simulink model "My_Design"  (R2024b)
settings: Solver=ode23t  StartTime=0.0  StopTime=0.5  RelTol=1e-3
libraries: powerlib_extras x16, spsThreePhaseBreakerLib x7, spsSeriesRLCBranchLib x6, spsLinearTransformerLib x6, spsCurrentMeasurementLib x6, fuzblock x3, simulink_extras x3, spsThreePhaseFaultLib x3, spsThreePhasePISectionLineLib x2, spsThreePhaseSourceLib x1, spsThreePhaseSeriesRLCLoadLib x1, spsThreePhaseTransformerTwoWindingsLib x1
settings Model: PauseTimes=0.2999  Creator=Isaac  LastModifiedBy=oppon
settings SolverCC: AlgebraicLoopSolver=TrustRegion
settings DataIOCC: ReturnWorkspaceOutputs=off
settings DebuggingCC: UnconnectedInputMsg=warning  UnconnectedOutputMsg=warning  UnconnectedLineMsg=warning  ArithmeticOperatorsInVariantConditions=warning
settings ModelReferenceCC: EnableRefExpFcnMdlSchedulingChecks=on
settings SFSimCC: CustomCodeUndefinedFunction=UseInterfaceOnly
settings RTWCC: GPUComputeCapability=3.5

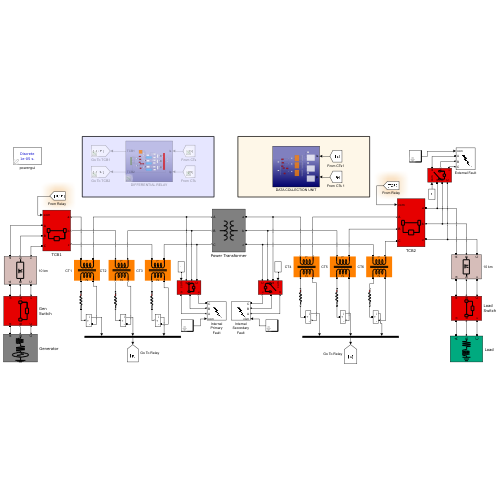
[thumbnail: Simulink's stored preview of the top-level diagram]
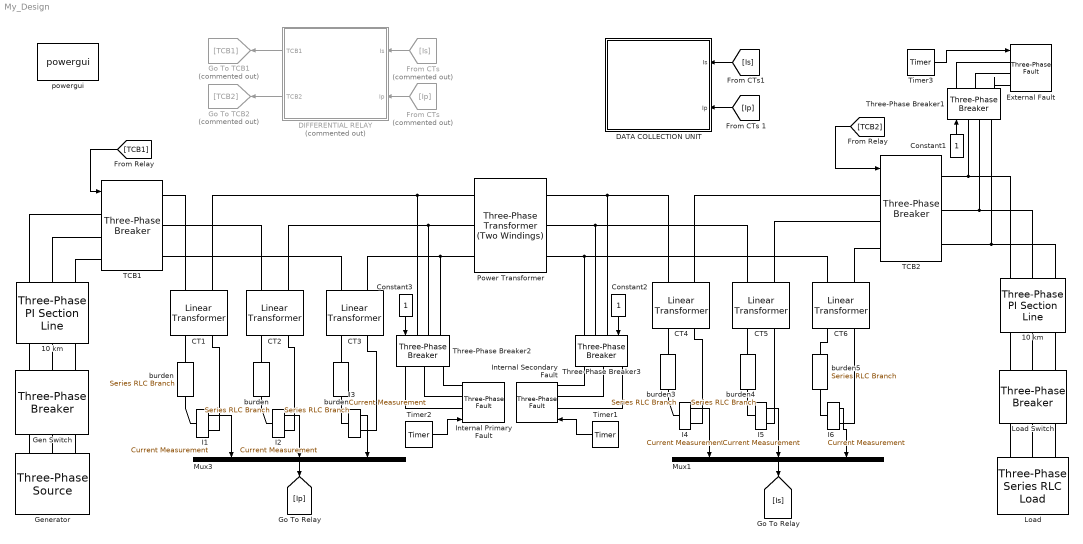
== system My_Design ==
  " burden " : spsSeriesRLCBranchLib/Series RLC Branch  LConnTagsString=__new0  RConnTagsString=__new0  BranchType=R  Resistance=1  Inductance=[]  SetiL0=off  InitialCurrent=0  Capacitance=[]  Setx0=off  InitialVoltage=0  Measurements=None
  10 km : spsThreePhasePISectionLineLib/Three-Phase PI Section Line  LConnTagsString=a|b|c  RConnTagsString=A|B|C  Length=10  Frequency=50  Resistances=[ 0.01273 0.3864]  Inductances="[ 0.9337e-3  4.1264e-3]"  Capacitances=[12.74e-9 7.751e-9]
  "10 km " : spsThreePhasePISectionLineLib/Three-Phase PI Section Line  LConnTagsString=a|b|c  RConnTagsString=A|B|C  Length=10  Frequency=50  Resistances=[ 0.01273 0.3864]  Inductances="[ 0.9337e-3  4.1264e-3]"  Capacitances=[12.74e-9 7.751e-9]
  CT1 : spsLinearTransformerLib/Linear Transformer  UNITS=pu  NominalPower=[ 25 50 ]  winding1=[12*(5/100) 0.001 0.04]  winding2=[5 0.001 0.04 ]  ThreeWindings=off  winding3=[ 315e3 0.002 0.08 ]  RmLm=[ 100 100 ]  Measurements=None  DataType=off
  CT2 : spsLinearTransformerLib/Linear Transformer  UNITS=pu  NominalPower=[ 25 50 ]  winding1=[12*(5/100) 0.001 0.04]  winding2=[5 0.001 0.04 ]  ThreeWindings=off  winding3=[ 315e3 0.002 0.08 ]  RmLm=[ 100 100 ]  Measurements=None  DataType=off
  CT3 : spsLinearTransformerLib/Linear Transformer  UNITS=pu  NominalPower=[ 25 50 ]  winding1=[12*(5/100) 0.001 0.04]  winding2=[5 0.001 0.04 ]  ThreeWindings=off  winding3=[ 315e3 0.002 0.08 ]  RmLm=[ 100 100 ]  Measurements=None  DataType=off
  CT4 : spsLinearTransformerLib/Linear Transformer  UNITS=pu  NominalPower=[ 25 50 ]  winding1=[14*(5/550) 0.001 0.04]  winding2=[5 0.001 0.04 ]  ThreeWindings=off  winding3=[ 315e3 0.002 0.08 ]  RmLm=[ 100 100 ]  Measurements=None  DataType=off
  CT5 : spsLinearTransformerLib/Linear Transformer  UNITS=pu  NominalPower=[ 25 50 ]  winding1=[14*(5/550) 0.001 0.04]  winding2=[5 0.001 0.04 ]  ThreeWindings=off  winding3=[ 315e3 0.002 0.08 ]  RmLm=[ 100 100 ]  Measurements=None  DataType=off
  CT6 : spsLinearTransformerLib/Linear Transformer  UNITS=pu  NominalPower=[ 25 50 ]  winding1=[14*(5/550) 0.001 0.04]  winding2=[5 0.001 0.04 ]  ThreeWindings=off  winding3=[ 315e3 0.002 0.08 ]  RmLm=[ 100 100 ]  Measurements=None  DataType=off
  Constant1 : Constant  OutDataTypeStr=boolean
  Constant2 : Constant  OutDataTypeStr=boolean
  Constant3 : Constant  OutDataTypeStr=boolean
  DATA COLLECTION UNIT : Subsystem
  DIFFERENTIAL RELAY : Subsystem  Commented=on
  External Fault : spsThreePhaseFaultLib/Three-Phase Fault  InitialStates=0  FaultA=on  FaultB=off  FaultC=off  GroundFault=on  SwitchTimes="[1/60  5/60]"  External=on  SwitchStatus=NaN  FaultResistance=0.001  GroundResistance=0.01  SnubberResistance=1e6  SnubberCapacitance=inf  Measurements=None
  From CTs : From  Commented=on  GotoTag=Is
  "From CTs " : From  Commented=on  GotoTag=Ip
  Gen Switch : spsThreePhaseBreakerLib/Three-Phase Breaker  InitialState=closed  SwitchA=off  SwitchB=off  SwitchC=off  SwitchTimes=[0.4/60 0.8/60 1/60 2.5/60]  External=off  BreakerResistance=0.001  SnubberResistance=1e6  SnubberCapacitance=inf  Measurements=None
  Generator : spsThreePhaseSourceLib/Three-Phase Source  InternalConnection=Yg  VoltagePhases=off  Voltage=161e3/sqrt(3)  PhaseAngle=0  Voltage_phases=[161e3 161e3 161e3]  PhaseAngles_phases=[0 -120 +120]  Frequency=50  NonIdealSource=on  SpecifyImpedance=on  Resistance=0.8929  Inductance=16.58e-3  ShortCircuitLevel=100e6  BaseVoltage=161e3/sqrt(3)  XRratio=2  BusType=swing  Pref=0  Qref=0  Prefabc=[10e3, 10e3, 10e3]  Qrefabc=[0, 0, 0]  Qmin=-inf  Qmax=inf
  Go To TCB1 : Goto  Commented=on  GotoTag=TCB1
  Go To TCB2 : Goto  Commented=on  GotoTag=TCB2
  I{1..6} (6 alike) : spsCurrentMeasurementLib/Current Measurement  Tag=PoWeRsYsTeMmEaSuReMeNt  PhasorSimulation=off  OutputType=Magnitude  PSBequivalent=0
      settings: AttributesFormatString=\n
  Internal Primary Fault : spsThreePhaseFaultLib/Three-Phase Fault  InitialStates=0  FaultA=on  FaultB=on  FaultC=on  GroundFault=off  SwitchTimes="[1/60  5/60]"  External=on  SwitchStatus=NaN  FaultResistance=0.001  GroundResistance=0.01  SnubberResistance=1e6  SnubberCapacitance=inf  Measurements=None
  Internal Secondary Fault : spsThreePhaseFaultLib/Three-Phase Fault  InitialStates=0  FaultA=on  FaultB=on  FaultC=on  GroundFault=on  SwitchTimes="[1/60  5/60]"  External=on  SwitchStatus=NaN  FaultResistance=0.001  GroundResistance=0.01  SnubberResistance=1e6  SnubberCapacitance=inf  Measurements=None
  Load : spsThreePhaseSeriesRLCLoadLib/Three-Phase Series RLC Load  LConnTagsString=A|B|C  Configuration=Y (grounded)  NominalVoltage=34.5e3  Vabc=[1e3 1e3 1e3]  Vabcp=[1e3 1e3 1e3]  NominalFrequency=50  UnbalancedPower=off  ActivePower=10e6  InductivePower=23e6  CapacitivePower=0  Pabc=[10e3 9e3 11e3]  QLabc=[100 90 110]  QCabc=[100 90 110]  Pabcp=[10e3 9e3 11e3]  QLabcp=[100 90 110]  QCabcp=[100 90 110]  Measurements=None  LoadType=constant Z
  Load Switch : spsThreePhaseBreakerLib/Three-Phase Breaker  InitialState=closed  SwitchA=off  SwitchB=off  SwitchC=off  SwitchTimes="[4/60  10/60]"  External=off  BreakerResistance=0.001  SnubberResistance=1e6  SnubberCapacitance=inf  Measurements=None
  Mux1 : Mux  Inputs=3
  Mux3 : Mux  Inputs=3
  Power Transformer : spsThreePhaseTransformerTwoWindingsLib/Three-Phase Transformer (Two Windings)  Winding1Connection=Yg  Winding2Connection=Yg  CoreType=Three-limb core (core-type)  SetSaturation=off  Hysteresis=off  DataFile='hysteresis'  SetInitialFlux=on  Measurements=All measurements (V I Fluxes)  UNITS=pu  NominalPower=[ 50e6 , 50 ]  Winding1=[1.61e+05 0.002 0.08]  Winding2=[34500 0.002 0.08]  Rm=500  Lm=1e6  L0=0.5  Saturation=[ 0,0 ; 0.015,1.2; 0.03,1.35; 0.06,1.5; 0.09,1.56; 0.12,1.572; 2.5e+12,1e+12]  InitialFluxes=[-0.291269118191543 0.0927265830204329 0.198559664112565]  BreakLoop=off  DiscreteSolver=Trapezoidal iterative  DataType=off  TransfoNumber=1
  TCB1 : spsThreePhaseBreakerLib/Three-Phase Breaker  InitialState=closed  SwitchA=off  SwitchB=off  SwitchC=off  SwitchTimes="[4/60  10/60]"  External=on  BreakerResistance=0.001  SnubberResistance=1e6  SnubberCapacitance=inf  Measurements=None
  TCB2 : spsThreePhaseBreakerLib/Three-Phase Breaker  InitialState=closed  SwitchA=off  SwitchB=off  SwitchC=off  SwitchTimes="[4/60  10/60]"  External=on  BreakerResistance=0.001  SnubberResistance=1e6  SnubberCapacitance=inf  Measurements=None
  Three-Phase Breaker1 : spsThreePhaseBreakerLib/Three-Phase Breaker  InitialState=open  SwitchA=on  SwitchB=on  SwitchC=on  SwitchTimes="[1/60  5/60]"  External=on  BreakerResistance=0.01  SnubberResistance=1e6  SnubberCapacitance=inf  Measurements=None
  Three-Phase Breaker2 : spsThreePhaseBreakerLib/Three-Phase Breaker  InitialState=closed  SwitchA=on  SwitchB=on  SwitchC=on  SwitchTimes="[1/60  5/60]"  External=on  BreakerResistance=0.01  SnubberResistance=1e6  SnubberCapacitance=inf  Measurements=None
  Three-Phase Breaker3 : spsThreePhaseBreakerLib/Three-Phase Breaker  InitialState=open  SwitchA=on  SwitchB=on  SwitchC=on  SwitchTimes="[1/60  5/60]"  External=on  BreakerResistance=0.01  SnubberResistance=1e6  SnubberCapacitance=inf  Measurements=None
  Timer1 : powerlib_extras/Control  Blocks/Timer  t=[0 0.3]  e=[0 1]
  Timer2 : powerlib_extras/Control  Blocks/Timer  t=[0 0.2]  e=[0 1]
  Timer3 : powerlib_extras/Control  Blocks/Timer  t=[0 0.4]  e=[0 1]
  burden{,3..5} (4 alike) : spsSeriesRLCBranchLib/Series RLC Branch  LConnTagsString=__new0  RConnTagsString=__new0  BranchType=R  Resistance=1  Inductance=[]  SetiL0=off  InitialCurrent=0  Capacitance=[]  Setx0=off  InitialVoltage=0  Measurements=None
  "burden " : spsSeriesRLCBranchLib/Series RLC Branch  LConnTagsString=__new0  RConnTagsString=__new0  BranchType=R  Resistance=1  Inductance=[]  SetiL0=off  InitialCurrent=0  Capacitance=[]  Setx0=off  InitialVoltage=0  Measurements=None
  powergui : sps_lib/powergui  Priority=1  SimulationMode=Discrete  SampleTime=1e-5  frequency=50  Iterations=50  frequencyindice=50  Pbase=100e6  ErrMax=1e-4  UnitsV=kV  UnitsW=MW  buscounter=0  FunctionMessages=off  echomessages=off  EnableUseOfTLC=off  CurrentSourceSwitches=off  DisableSnubberDevices=off  DisableRonSwitches=off  DisableVfSwitches=off  DisplayEquations=off  AutomaticDiscreteSolvers=off  SolverType=Tustin/Backward Euler (TBE)  Interpol=off  ExternalGateDelay=off  methode=off  Ts=100  x0status=blocks  SPID=off  SwTol=0  HookPort=off  NonlinearTolerance=1e-4  nMaxIteration=100  ContinueOnMaxIteration=off  RestoreLinks=warning  ResistiveCurrentMeasurement=off  Frange=[0:2:500]  Ylog=off  Xlog=on  ShowGrid=off  save=off  variable=ZData  structure=0  ZoomFFT=on  StartTime=0.0  cycles=1  DisplayStyle=1  fundamental=60  FreqAxis=off  MaxFrequency=1000  frequencyindicesteady=1  RmsSteady=1  display=off
  wires:
  Constant3/1 -> Three-Phase Breaker2/1
  Timer3/1 -> External Fault/1
  I4/1 -> Mux1/1
  Constant1/1 -> Three-Phase Breaker1/1
  I1/1 -> Mux3/1
  Mux1/1 -> [Is]
  [TCB1] -> TCB1/1
  Mux3/1 -> [Ip]
  I6/1 -> Mux1/3
  Timer1/1 -> Internal Secondary Fault/1
  [TCB2] -> TCB2/1
  I2/1 -> Mux3/2
  Timer2/1 -> Internal Primary Fault/1
  I5/1 -> Mux1/2
  Constant2/1 -> Three-Phase Breaker3/1
  DIFFERENTIAL RELAY/1(TCB1) -> Go To TCB1/1
  I3/1 -> Mux3/3
  "From CTs "/1 -> DIFFERENTIAL RELAY/2(Ip)
  From CTs/1 -> DIFFERENTIAL RELAY/1(Is)
  DIFFERENTIAL RELAY/2(TCB2) -> Go To TCB2/1
  [Is] -> DATA COLLECTION UNIT/1(Is)
  [Ip] -> DATA COLLECTION UNIT/2(Ip)
  connections:
  Three-Phase Breaker1/LConn1 -- TCB2/RConn1 -- "10 km "/LConn1
  Power Transformer/RConn1 -- CT4/LConn2 -- Three-Phase Breaker3/LConn1
  Three-Phase Breaker2/LConn1 -- CT1/LConn1 -- Power Transformer/LConn1
  Power Transformer/RConn3 -- CT6/LConn2 -- Three-Phase Breaker3/LConn3
  Three-Phase Breaker2/LConn2 -- CT2/LConn1 -- Power Transformer/LConn2
  "10 km "/LConn2 -- TCB2/RConn2 -- Three-Phase Breaker1/LConn2
  "10 km "/LConn3 -- TCB2/RConn3 -- Three-Phase Breaker1/LConn3
  Power Transformer/RConn2 -- CT5/LConn2 -- Three-Phase Breaker3/LConn2
  Three-Phase Breaker2/LConn3 -- CT3/LConn1 -- Power Transformer/LConn3
  10 km/RConn2 -- TCB1/LConn2
  Three-Phase Breaker1/RConn2 -- External Fault/LConn2
  10 km/RConn3 -- TCB1/LConn3
  burden/RConn1 -- I1/LConn1
  Three-Phase Breaker3/RConn3 -- Internal Secondary Fault/LConn3
  CT3/LConn2 -- TCB1/RConn3
  burden3/LConn1 -- CT4/RConn2
  Three-Phase Breaker1/RConn3 -- External Fault/LConn3
  CT4/LConn1 -- TCB2/LConn1
  I6/RConn1 -- CT6/RConn1
  burden4/LConn1 -- CT5/RConn2
  burden5/RConn1 -- I6/LConn1
  burden5/LConn1 -- CT6/RConn2
  CT6/LConn1 -- TCB2/LConn3
  CT2/LConn2 -- TCB1/RConn2
  "10 km "/RConn1 -- Load Switch/LConn1
  "burden "/LConn1 -- CT2/RConn2
  Gen Switch/LConn1 -- Generator/RConn1
  I1/RConn1 -- CT1/RConn1
  I3/RConn1 -- CT3/RConn1
  I4/RConn1 -- CT4/RConn1
  "10 km "/RConn2 -- Load Switch/LConn2
  "10 km "/RConn3 -- Load Switch/LConn3
  Three-Phase Breaker2/RConn3 -- Internal Primary Fault/LConn3
  " burden "/LConn1 -- CT3/RConn2
  Three-Phase Breaker2/RConn2 -- Internal Primary Fault/LConn2
  burden/LConn1 -- CT1/RConn2
  Load/LConn3 -- Load Switch/RConn3
  10 km/LConn3 -- Gen Switch/RConn3
  Gen Switch/LConn3 -- Generator/RConn3
  Gen Switch/LConn2 -- Generator/RConn2
  10 km/LConn1 -- Gen Switch/RConn1
  10 km/RConn1 -- TCB1/LConn1
  Load Switch/RConn1 -- Load/LConn1
  Three-Phase Breaker1/RConn1 -- External Fault/LConn1
  CT5/RConn1 -- I5/RConn1
  burden3/RConn1 -- I4/LConn1
  Three-Phase Breaker3/RConn1 -- Internal Secondary Fault/LConn1
  burden4/RConn1 -- I5/LConn1
  "burden "/RConn1 -- I2/LConn1
  Three-Phase Breaker3/RConn2 -- Internal Secondary Fault/LConn2
  CT5/LConn1 -- TCB2/LConn2
  Load/LConn2 -- Load Switch/RConn2
  Three-Phase Breaker2/RConn1 -- Internal Primary Fault/LConn1
  " burden "/RConn1 -- I3/LConn1
  10 km/LConn2 -- Gen Switch/RConn2
  CT2/RConn1 -- I2/RConn1
  CT1/LConn2 -- TCB1/RConn1

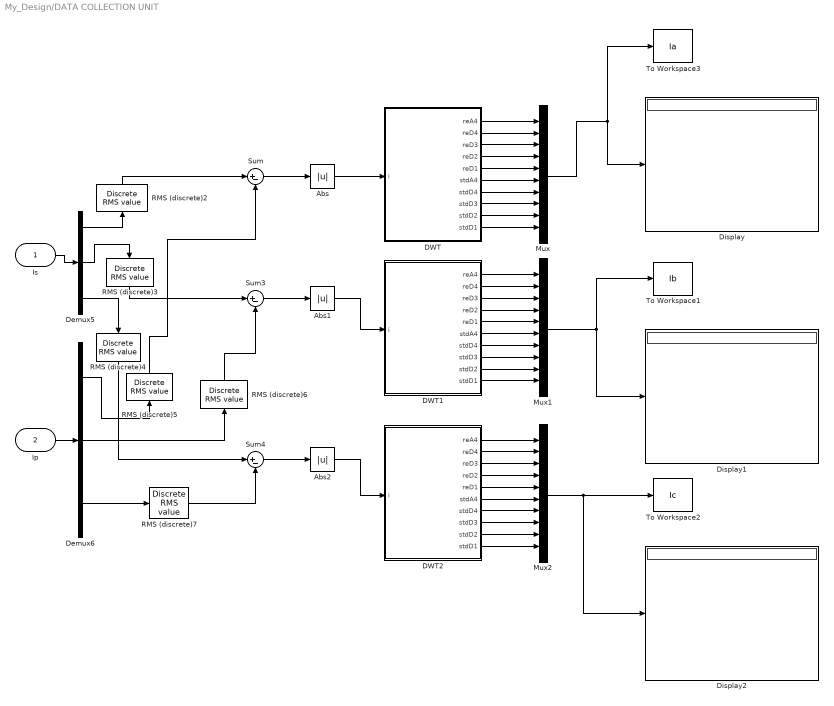
== system My_Design/DATA COLLECTION UNIT ==
  Is : Inport
  Ip : Inport  Port=2
  Abs : Abs  SaturateOnIntegerOverflow=off
  Abs1 : Abs  SaturateOnIntegerOverflow=off
  Abs2 : Abs  SaturateOnIntegerOverflow=off
  DWT : MATLAB Function  TreatAsAtomicUnit=on
  DWT1 : MATLAB Function  TreatAsAtomicUnit=on
  DWT2 : MATLAB Function  TreatAsAtomicUnit=on
  Demux5 : Demux  Outputs=3
  Demux6 : Demux  Outputs=3
  Display : Display
  Display1 : Display
  Display2 : Display
  Mux : Mux  Inputs=10
  Mux1 : Mux  Inputs=10
  Mux2 : Mux  Inputs=10
  RMS (discrete){2..7} (6 alike) : powerlib_extras/Discrete Measurements/Discrete  RMS value  Freq=50  Mag_Init=0  Ts=0.001
  Sum : Sum  Inputs=|+-
  Sum3 : Sum  Inputs=|+-
  Sum4 : Sum  Inputs=|+-
  To Workspace1 : ToWorkspace  VariableName=Ib  SampleTime=-1
      settings: Save2DSignal=2-D array (concatenate along first dimension)
  To Workspace2 : ToWorkspace  VariableName=Ic  SampleTime=-1
      settings: Save2DSignal=2-D array (concatenate along first dimension)
  To Workspace3 : ToWorkspace  VariableName=Ia  SampleTime=-1
      settings: Save2DSignal=2-D array (concatenate along first dimension)
  wires:
  Demux6/1 -> RMS (discrete)5/1
  Demux5/2 -> RMS (discrete)3/1
  Demux6/2 -> RMS (discrete)6/1
  Demux5/1 -> RMS (discrete)2/1
  Demux5/3 -> RMS (discrete)4/1
  Demux6/3 -> RMS (discrete)7/1
  Is/1 -> Demux5/1
  Ip/1 -> Demux6/1
  RMS (discrete)2/1 -> Sum/1
  RMS (discrete)5/1 -> Sum/2
  RMS (discrete)3/1 -> Sum3/1
  RMS (discrete)4/1 -> Sum4/1
  RMS (discrete)6/1 -> Sum3/2
  RMS (discrete)7/1 -> Sum4/2
  Sum/1 -> Abs/1
  Sum3/1 -> Abs1/1
  Sum4/1 -> Abs2/1
  Abs/1 -> DWT/1(i)
  DWT/1(reA4) -> Mux/1
  DWT/2(reD4) -> Mux/2
  DWT/3(reD3) -> Mux/3
  DWT/4(reD2) -> Mux/4
  DWT/5(reD1) -> Mux/5
  DWT/6(stdA4) -> Mux/6
  DWT/7(stdD4) -> Mux/7
  DWT/8(stdD3) -> Mux/8
  DWT/9(stdD2) -> Mux/9
  DWT/10(stdD1) -> Mux/10
  Mux/1 -> To Workspace3/1, Display/1
  DWT1/6(stdA4) -> Mux1/6
  DWT1/5(reD1) -> Mux1/5
  DWT1/2(reD4) -> Mux1/2
  DWT1/1(reA4) -> Mux1/1
  DWT1/4(reD2) -> Mux1/4
  DWT1/10(stdD1) -> Mux1/10
  DWT1/9(stdD2) -> Mux1/9
  DWT1/3(reD3) -> Mux1/3
  DWT1/8(stdD3) -> Mux1/8
  DWT1/7(stdD4) -> Mux1/7
  DWT2/6(stdA4) -> Mux2/6
  DWT2/5(reD1) -> Mux2/5
  DWT2/2(reD4) -> Mux2/2
  DWT2/1(reA4) -> Mux2/1
  DWT2/4(reD2) -> Mux2/4
  DWT2/10(stdD1) -> Mux2/10
  DWT2/9(stdD2) -> Mux2/9
  DWT2/3(reD3) -> Mux2/3
  DWT2/8(stdD3) -> Mux2/8
  DWT2/7(stdD4) -> Mux2/7
  Abs2/1 -> DWT2/1(i)
  Abs1/1 -> DWT1/1(i)
  Mux2/1 -> Display2/1, To Workspace2/1
  Mux1/1 -> Display1/1, To Workspace1/1

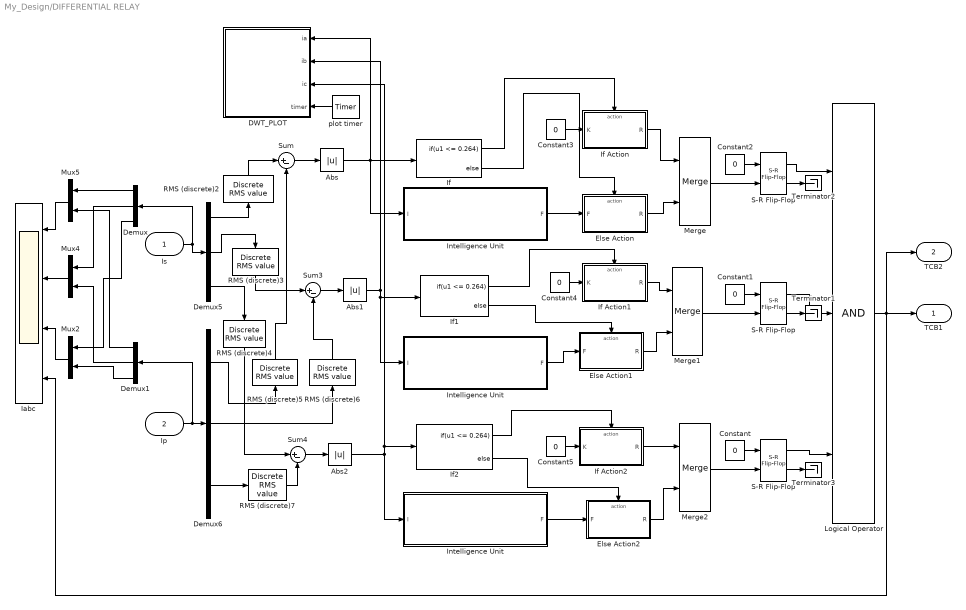
== system My_Design/DIFFERENTIAL RELAY ==
  Is : Inport
  Ip : Inport  Port=2
  " Logical Operator" : Logic  Inputs=3  AllPortsSameDT=off  OutDataTypeStr=boolean
  Abs : Abs  SaturateOnIntegerOverflow=off
  Abs1 : Abs  SaturateOnIntegerOverflow=off
  Abs2 : Abs  SaturateOnIntegerOverflow=off
  Constant{,1..5} (6 alike) : Constant  Value=0  OutDataTypeStr=boolean
  DWT_PLOT : MATLAB Function  TreatAsAtomicUnit=on
  Demux{,1,5..6} (4 alike) : Demux  Outputs=3
  Else Action : Subsystem  TreatAsAtomicUnit=on
  Else Action1 : Subsystem  TreatAsAtomicUnit=on
  Else Action2 : Subsystem  TreatAsAtomicUnit=on
  Iabc : Scope  NumInputPorts=4
  If : If  IfExpression=u1 <= 0.264
  If Action : Subsystem  TreatAsAtomicUnit=on
  If Action1 : Subsystem  TreatAsAtomicUnit=on
  If Action2 : Subsystem  TreatAsAtomicUnit=on
  If1 : If  IfExpression=u1 <= 0.264
  If2 : If  IfExpression=u1 <= 0.264
  Intelligence Unit : Subsystem
  "Intelligence Unit " : Subsystem
  "Intelligence Unit  " : Subsystem
  Merge : Merge
  Merge1 : Merge
  Merge2 : Merge
  Mux2 : Mux  Inputs=2
  Mux4 : Mux  Inputs=2
  Mux5 : Mux  Inputs=2
  RMS (discrete){2..7} (6 alike) : powerlib_extras/Discrete Measurements/Discrete  RMS value  Freq=50  Mag_Init=0  Ts=0.001
  "S-R Flip-Flop " : simulink_extras/Flip Flops/S-R Flip-Flop  initial_condition=1
  "S-R Flip-Flop  " : simulink_extras/Flip Flops/S-R Flip-Flop  initial_condition=1
  S-R Flip-Flop : simulink_extras/Flip Flops/S-R Flip-Flop  initial_condition=1
  Sum : Sum  Inputs=|+-
  Sum3 : Sum  Inputs=|+-
  Sum4 : Sum  Inputs=|+-
  Terminator1 : Terminator
  Terminator2 : Terminator
  Terminator3 : Terminator
  plot timer : powerlib_extras/Control  Blocks/Timer  t=[0 0.299999999999]  e=[0 1]
  TCB1 : Outport  VectorParamsAs1DForOutWhenUnconnected=off
  TCB2 : Outport  Port=2  VectorParamsAs1DForOutWhenUnconnected=off
  wires:
  "S-R Flip-Flop  "/1 -> " Logical Operator"/3
  Constant/1 -> "S-R Flip-Flop  "/1
  "S-R Flip-Flop  "/2 -> Terminator3/1
  "S-R Flip-Flop "/2 -> Terminator1/1
  Constant1/1 -> "S-R Flip-Flop "/1
  Constant2/1 -> S-R Flip-Flop/1
  S-R Flip-Flop/2 -> Terminator2/1
  S-R Flip-Flop/1 -> " Logical Operator"/1
  "S-R Flip-Flop "/1 -> " Logical Operator"/2
  Demux6/1 -> RMS (discrete)5/1
  Demux5/2 -> RMS (discrete)3/1
  Demux6/2 -> RMS (discrete)6/1
  Demux5/1 -> RMS (discrete)2/1
  Demux5/3 -> RMS (discrete)4/1
  Demux6/3 -> RMS (discrete)7/1
  If1/1 -> If Action1/Action
  If/2 -> Else Action/Action
  If1/2 -> Else Action1/Action
  Intelligence Unit/1(F) -> Else Action/1(F)
  Else Action/1(R) -> Merge/2
  If Action/1(R) -> Merge/1
  Merge/1 -> S-R Flip-Flop/2
  Merge1/1 -> "S-R Flip-Flop "/2
  Merge2/1 -> "S-R Flip-Flop  "/2
  Constant3/1 -> If Action/1(K)
  Constant4/1 -> If Action1/1(K)
  Demux1/2 -> Mux4/2
  Demux1/3 -> Mux2/2
  Mux5/1 -> Iabc/1
  Demux1/1 -> Mux5/2
  Demux/1 -> Mux5/1
  Mux2/1 -> Iabc/3
  Demux/2 -> Mux4/1
  Mux4/1 -> Iabc/2
  Demux/3 -> Mux2/1
  Is/1 -> Demux/1, Demux5/1
  " Logical Operator"/1 -> Iabc/4, TCB2/1, TCB1/1
  Ip/1 -> Demux1/1, Demux6/1
  RMS (discrete)2/1 -> Sum/1
  RMS (discrete)5/1 -> Sum/2
  RMS (discrete)3/1 -> Sum3/1
  RMS (discrete)4/1 -> Sum4/1
  RMS (discrete)6/1 -> Sum3/2
  RMS (discrete)7/1 -> Sum4/2
  Sum/1 -> Abs/1
  Abs/1 -> DWT_PLOT/1(ia), Intelligence Unit/1(I), If/1
  Sum3/1 -> Abs1/1
  Abs1/1 -> "Intelligence Unit "/1(I), If1/1, DWT_PLOT/2(ib)
  Sum4/1 -> Abs2/1
  Abs2/1 -> DWT_PLOT/3(ic), If2/1, "Intelligence Unit  "/1(I)
  If/1 -> If Action/Action
  "Intelligence Unit  "/1(F) -> Else Action2/1(F)
  If Action1/1(R) -> Merge1/1
  "Intelligence Unit "/1(F) -> Else Action1/1(F)
  Else Action1/1(R) -> Merge1/2
  Constant5/1 -> If Action2/1(K)
  If Action2/1(R) -> Merge2/1
  If2/1 -> If Action2/Action
  If2/2 -> Else Action2/Action
  Else Action2/1(R) -> Merge2/2
  plot timer/1 -> DWT_PLOT/4(timer)

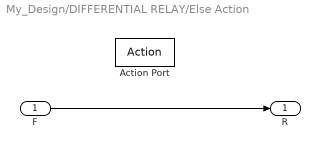
== system My_Design/DIFFERENTIAL RELAY/Else Action ==
  F : Inport
  Action Port : ActionPort  ActionPortLabel=else
  R : Outport  VectorParamsAs1DForOutWhenUnconnected=off
  wires:
  F/1 -> R/1

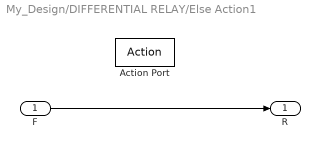
== system My_Design/DIFFERENTIAL RELAY/Else Action1 ==
  F : Inport
  Action Port : ActionPort  ActionPortLabel=else
  R : Outport  VectorParamsAs1DForOutWhenUnconnected=off
  wires:
  F/1 -> R/1

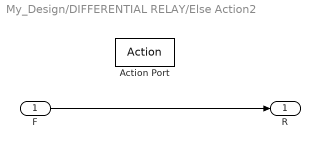
== system My_Design/DIFFERENTIAL RELAY/Else Action2 ==
  F : Inport
  Action Port : ActionPort  ActionPortLabel=else
  R : Outport  VectorParamsAs1DForOutWhenUnconnected=off
  wires:
  F/1 -> R/1

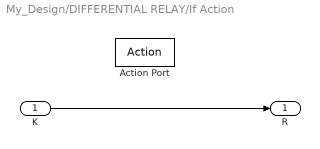
== system My_Design/DIFFERENTIAL RELAY/If Action ==
  K : Inport
  Action Port : ActionPort  ActionPortLabel=if(u1 <= 0.264)
  R : Outport
  wires:
  K/1 -> R/1

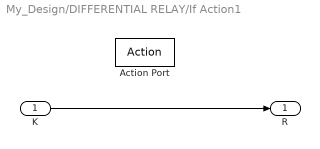
== system My_Design/DIFFERENTIAL RELAY/If Action1 ==
  K : Inport
  Action Port : ActionPort  ActionPortLabel=if(u1 <= 0.264)
  R : Outport
  wires:
  K/1 -> R/1

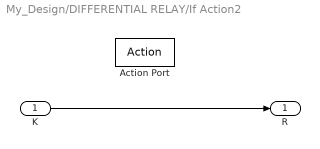
== system My_Design/DIFFERENTIAL RELAY/If Action2 ==
  K : Inport
  Action Port : ActionPort  ActionPortLabel=if(u1 <= 0.264)
  R : Outport
  wires:
  K/1 -> R/1

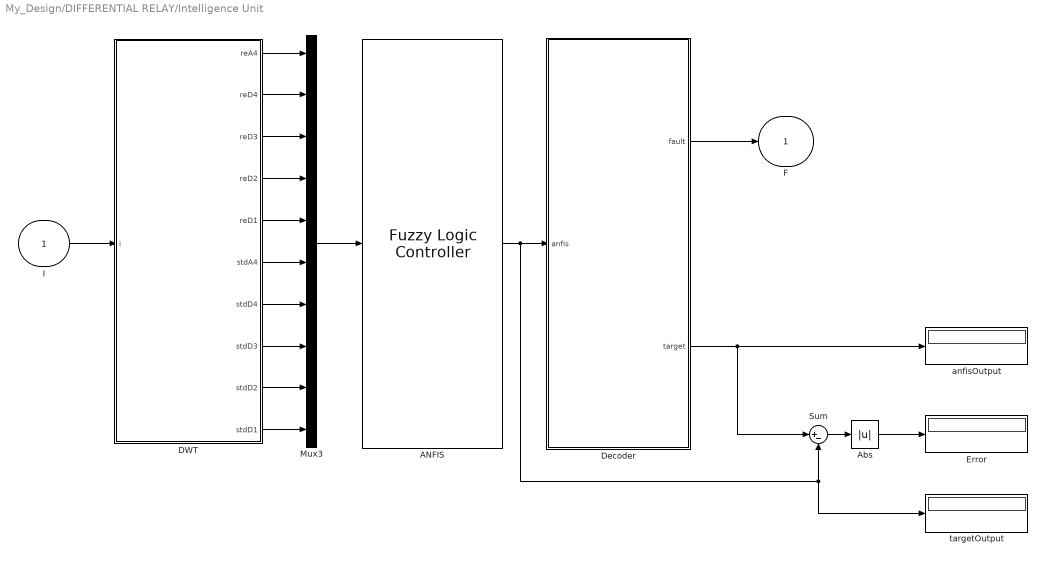
== system My_Design/DIFFERENTIAL RELAY/Intelligence Unit ==
  I : Inport
  ANFIS : fuzblock/Fuzzy Logic  Controller  FIS='classifier.fis'  OutputSampleNumber=101  DataType=double  FuzzifiedInputs=off  RuleFiringStrengths=off  RuleOutputs=off  AggregatedOutputs=off  SimulateUsing=Interpreted execution  OutOfRangeInputValueMessage=warning  NoRuleFiredMessage=warning  EmptyOutputFuzzySetMessage=warning
  Abs : Abs  SaturateOnIntegerOverflow=off
  DWT : MATLAB Function  TreatAsAtomicUnit=on
  Decoder : MATLAB Function  TreatAsAtomicUnit=on
  Error : Display
  Mux3 : Mux  Inputs=10
  Sum : Sum  Inputs=|+-
  anfisOutput : Display
  targetOutput : Display
  F : Outport  VectorParamsAs1DForOutWhenUnconnected=off
  wires:
  ANFIS/1 -> targetOutput/1, Sum/2, Decoder/1(anfis)
  I/1 -> DWT/1(i)
  Mux3/1 -> ANFIS/1
  DWT/1(reA4) -> Mux3/1
  DWT/2(reD4) -> Mux3/2
  DWT/3(reD3) -> Mux3/3
  DWT/4(reD2) -> Mux3/4
  DWT/5(reD1) -> Mux3/5
  DWT/6(stdA4) -> Mux3/6
  DWT/7(stdD4) -> Mux3/7
  DWT/8(stdD3) -> Mux3/8
  DWT/9(stdD2) -> Mux3/9
  DWT/10(stdD1) -> Mux3/10
  Decoder/1(fault) -> F/1
  Decoder/2(target) -> Sum/1, anfisOutput/1
  Sum/1 -> Abs/1
  Abs/1 -> Error/1

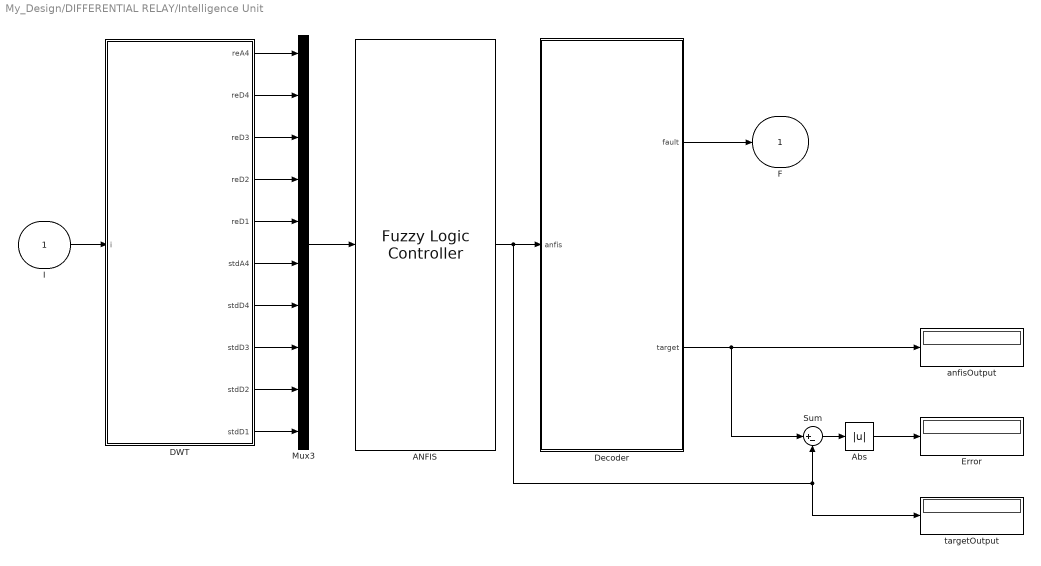
== system My_Design/DIFFERENTIAL RELAY/Intelligence Unit  ==
  I : Inport
  ANFIS : fuzblock/Fuzzy Logic  Controller  FIS='classifier.fis'  OutputSampleNumber=101  DataType=double  FuzzifiedInputs=off  RuleFiringStrengths=off  RuleOutputs=off  AggregatedOutputs=off  SimulateUsing=Interpreted execution  OutOfRangeInputValueMessage=warning  NoRuleFiredMessage=warning  EmptyOutputFuzzySetMessage=warning
  Abs : Abs  SaturateOnIntegerOverflow=off
  DWT : MATLAB Function  TreatAsAtomicUnit=on
  Decoder : MATLAB Function  TreatAsAtomicUnit=on
  Error : Display
  Mux3 : Mux  Inputs=10
  Sum : Sum  Inputs=|+-
  anfisOutput : Display
  targetOutput : Display
  F : Outport  VectorParamsAs1DForOutWhenUnconnected=off
  wires:
  Abs/1 -> Error/1
  Sum/1 -> Abs/1
  Decoder/2(target) -> anfisOutput/1, Sum/1
  Decoder/1(fault) -> F/1
  DWT/10(stdD1) -> Mux3/10
  DWT/9(stdD2) -> Mux3/9
  DWT/8(stdD3) -> Mux3/8
  DWT/7(stdD4) -> Mux3/7
  DWT/6(stdA4) -> Mux3/6
  DWT/5(reD1) -> Mux3/5
  DWT/4(reD2) -> Mux3/4
  DWT/3(reD3) -> Mux3/3
  DWT/2(reD4) -> Mux3/2
  DWT/1(reA4) -> Mux3/1
  Mux3/1 -> ANFIS/1
  I/1 -> DWT/1(i)
  ANFIS/1 -> Decoder/1(anfis), Sum/2, targetOutput/1

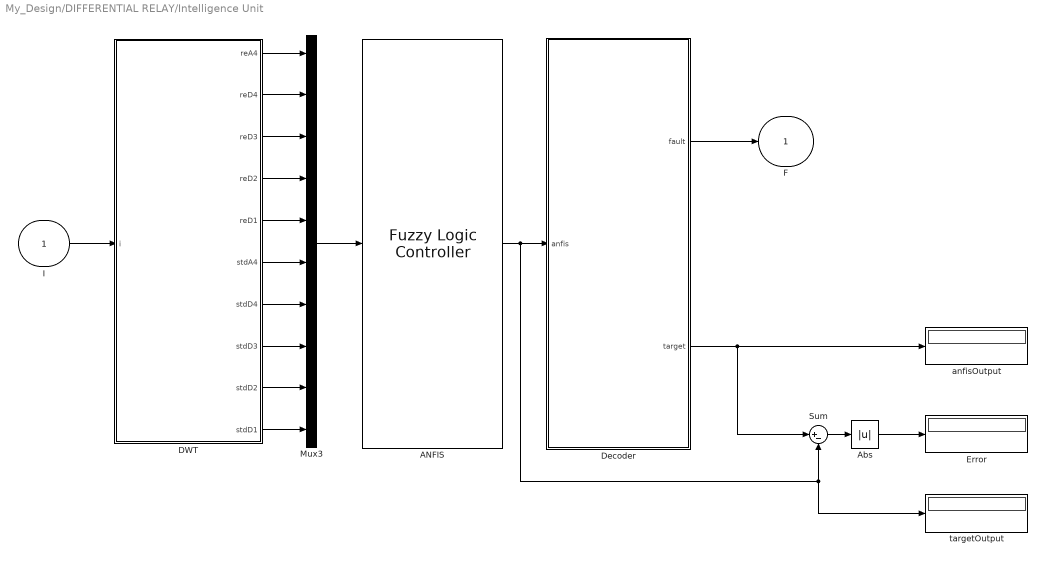
== system My_Design/DIFFERENTIAL RELAY/Intelligence Unit   ==
  I : Inport
  ANFIS : fuzblock/Fuzzy Logic  Controller  FIS='classifier.fis'  OutputSampleNumber=101  DataType=double  FuzzifiedInputs=off  RuleFiringStrengths=off  RuleOutputs=off  AggregatedOutputs=off  SimulateUsing=Interpreted execution  OutOfRangeInputValueMessage=warning  NoRuleFiredMessage=warning  EmptyOutputFuzzySetMessage=warning
  Abs : Abs  SaturateOnIntegerOverflow=off
  DWT : MATLAB Function  TreatAsAtomicUnit=on
  Decoder : MATLAB Function  TreatAsAtomicUnit=on
  Error : Display
  Mux3 : Mux  Inputs=10
  Sum : Sum  Inputs=|+-
  anfisOutput : Display
  targetOutput : Display
  F : Outport  VectorParamsAs1DForOutWhenUnconnected=off
  wires:
  ANFIS/1 -> targetOutput/1, Sum/2, Decoder/1(anfis)
  I/1 -> DWT/1(i)
  Mux3/1 -> ANFIS/1
  DWT/1(reA4) -> Mux3/1
  DWT/2(reD4) -> Mux3/2
  DWT/3(reD3) -> Mux3/3
  DWT/4(reD2) -> Mux3/4
  DWT/5(reD1) -> Mux3/5
  DWT/6(stdA4) -> Mux3/6
  DWT/7(stdD4) -> Mux3/7
  DWT/8(stdD3) -> Mux3/8
  DWT/9(stdD2) -> Mux3/9
  DWT/10(stdD1) -> Mux3/10
  Decoder/1(fault) -> F/1
  Decoder/2(target) -> Sum/1, anfisOutput/1
  Sum/1 -> Abs/1
  Abs/1 -> Error/1

== matlab function My_Design/DIFFERENTIAL RELAY/Intelligence Unit/Decoder ==
  data: anfis input; fault output; target output
function [fault, target] = DECODE(anfis)
%% INTERPRETATING THE RESULTS
%{
    The faults were representated numerically during the preprocessing
    state in Python. This was the represatation
    0 - Inrush condition / Transient current
    1 - Line faultt
    2 - Ground fault
    3 - normal condition / Healthy
%}
%% Give a tolerance of 10 for all faults since it is a practical system
persistent Faulttol;
if isempty(Faulttol)
    Faulttol = 0;
end
target = round(anfis);
if target == 0
    fault = false;
    condition = 'C: External Fault';
    disp(condition);
elseif target == 1
    condition = 'C: Ground Fault';
    disp(condition);
    fault = true;
elseif target == 2
    condition = 'C: Inrush Currents';
    disp(condition);
    fault = false;
elseif target == 3
    condition = 'C: Line Fault';
    disp(condition);
    fault = true;
else
    condition = 'C: Healthy';
    disp(condition);
    fault = false;
end

== matlab function My_Design/DIFFERENTIAL RELAY/Intelligence Unit  /DWT ==
  settings: updateMethod=DISCRETE  sampleTime=1e-5
  data: i input; reA4 output; reD4 output; reD3 output; reD2 output; reD1 output; stdA4 output; stdD4 output; stdD3 output; stdD2 output; stdD1 output
function [reA4,reD4,reD3,reD2, reD1,stdA4,stdD4,stdD3,stdD2,stdD1] = DWT(i)
%% CONVERT INPUT DISCRETE SAMPLES TO a 1-D SIGNAL
persistent I;
if isempty(I)
    I = i;
else
    I = [I; i];
end
%%
%% GET 1-D DISCRETE SIGNAL DIRECTLY FROM SAVED FAULTS
[CI,LI] = wavedec(I,4,'db4');
A4 = appcoef(CI,LI,'db4',4);
D4 = detcoef(CI,LI,4);
D3 = detcoef(CI,LI,3);
D2 = detcoef(CI,LI,2);
D1 = detcoef(CI,LI,1);
%% STATISTICAL AND RMS CALCULATIONS
Ej_A4 = sum(A4.^2);
Ej_D4 = sum(D4.^2);
Ej_D3 = sum(D3.^2);
Ej_D2 = sum(D2.^2);
Ej_D1 = sum(D1.^2);
E_total = Ej_A4 + Ej_D4 + Ej_D3 + Ej_D2 + Ej_D1;
reA4 = Ej_A4 / E_total;
reD4 = Ej_D4 / E_total;
reD3 = Ej_D3 / E_total;
reD2 = Ej_D2 / E_total;
reD1 = Ej_D1 / E_total;
stdA4 = std(A4);
stdD4 = std(D4);
stdD3 = std(D3);
stdD2 = std(D2);
stdD1 = std(D1);
end

== matlab function My_Design/DIFFERENTIAL RELAY/Intelligence Unit  /Decoder ==
  data: anfis input; fault output; target output
function [fault, target] = DECODE(anfis)
%% INTERPRETATING THE RESULTS
%{
    The faults were representated numerically during the preprocessing
    state in Python. This was the represatation
    0 - Inrush condition / Transient current
    1 - Line faultt
    2 - Ground fault
    3 - normal condition / Healthy
%}
%% Give a tolerance of 10 for all faults since it is a practical system
persistent Faulttol;
if isempty(Faulttol)
    Faulttol = 0;
end
target = round(anfis);
if target == 0
    fault = false;
    condition = 'C: External Fault';
    disp(condition);
elseif target == 1
    condition = 'C: Ground Fault';
    disp(condition);
    fault = true;
elseif target == 2
    condition = 'C: Inrush Currents';
    disp(condition);
    fault = false;
elseif target == 3
    condition = 'C: Line Fault';
    disp(condition);
    fault = true;
else
    condition = 'C: Healthy';
    disp(condition);
    fault = false;
end

== matlab function My_Design/DIFFERENTIAL RELAY/DWT_PLOT ==
  settings: updateMethod=DISCRETE  sampleTime=1e-5
  data: ia input; ib input; ic input; timer input
function PLOT(ia, ib, ic, timer)
    %% Declare variables
    persistent Ia;
    persistent Ib;
    persistent Ic;
    
    if round(timer) == 1
        %% INITIALIZE  AND CONVERT INPUT DISCRETE SAMPLES TO a 1-D SIGNAL
        if isempty(Ia)
            Ia = ia;
        else
            Ia = [Ia; ia];
        end
        if isempty(Ib)
            Ib = ib;
        else
            Ib = [Ib; ib];
        end
        if isempty(Ic)
            Ic = ic;
        else
            Ic = [Ic; ic];
        end
    
        %% PHASE A - decompose Ia signal
        [CIa,LIa] = wavedec(Ia,4,'db4');
        A4_Ia = appcoef(CIa,LIa,'db4',4);
        D4_Ia = detcoef(CIa,LIa,4);
        D3_Ia = detcoef(CIa,LIa,3);
        D2_Ia = detcoef(CIa,LIa,2);
        D1_Ia = detcoef(CIa,LIa,1);
        %% PHASE B - decompose Ib signal
        [CIb,LIb] = wavedec(Ib,4,'db4');
        A4_Ib = appcoef(CIb,LIb,'db4',4);
        D4_Ib = detcoef(CIb,LIb,4);
        D3_Ib = detcoef(CIb,LIb,3);
        D2_Ib = detcoef(CIb,LIb,2);
        D1_Ib = detcoef(CIb,LIb,1);
        %% PHASE C - decompose Ic signal
        [CIc,LIc] = wavedec(Ic,4,'db4');
        A4_Ic = appcoef(CIc,LIc,'db4',4);
        D4_Ic = detcoef(CIc,LIc,4);
        D3_Ic = detcoef(CIc,LIc,3);
        D2_Ic = detcoef(CIc,LIc,2);
        D1_Ic = detcoef(CIc,LIc,1);
    
        %% PLOT RESULTS
        figure('Name','DWT Decomposition','NumberTitle','off', 'Color',[1 1 1]);
        subplot(3,2,1);
        plot(Ia, 'r', 'LineWidth',1); hold on;
        plot(Ib, 'b', 'LineWidth',1); hold on;
        plot(Ic, 'g', 'LineWidth',1); hold off;
        xlabel({'Number of samples','(a) Differential Signal'},'FontWeight','bold');
        ylabel({'Magnitude'},'FontWeight','bold');
        leg = legend('show', 'Ia', 'Ib', 'Ic');
        set(leg,'Units','pixels',...
        'Orientation','vertical',...
        'location', 'northwest',...
        'Interpreter','none',...
        'FontSize',8,...
        'EdgeColor',[1 1 1]);
        %
        subplot(3,2,2);
        plot(A4_Ia, 'r', 'LineWidth',1); hold on;
        plot(A4_Ib, 'b', 'LineWidth',1); hold on;
        plot(A4_Ic, 'g', 'LineWidth',1); hold off;
        xlabel({'Number of samples','(b) A4 Coefficient'},'FontWeight','bold');
        ylabel({'Magnitude'},'FontWeight','bold');
        leg = legend('show', 'Ia', 'Ib', 'Ic');
        set(leg,'Units','pixels',...
        'Orientation','vertical',...
        'location', 'northwest',...
        'Interpreter','none',...
        'FontSize',8,...
        'EdgeColor',[1 1 1]);
        %
        subplot(3,2,3);
        plot(D4_Ia, 'r'); hold on;
        plot(D4_Ib, 'b'); hold on;
        plot(D4_Ic, 'g'); hold off;
        xlabel({'Number of samples','(c) D4 Coefficient'},'FontWeight','bold');
        ylabel({'Magnitude'},'FontWeight','bold');
        leg = legend('show', 'Ia', 'Ib', 'Ic');
        set(leg,'Units','pixels',...
        'Orientation','vertical',...
        'location', 'northwest',...
        'Interpreter','none',...
        'FontSize',8,...
        'EdgeColor',[1 1 1]);
        %
        subplot(3,2,4);
        plot(D3_Ia, 'r'); hold on;
        plot(D3_Ib, 'b'); hold on;
        plot(D3_Ic, 'g'); hold off;
        xlabel({'Number of samples','(d) D3 Coefficient'},'FontWeight','bold');
        ylabel({'Magnitude'},'FontWeight','bold');
        leg = legend('show', 'Ia', 'Ib', 'Ic');
        set(leg,'Units','pixels',...
        'Orientation','vertical',...
        'location', 'northwest',...
        'Interpreter','none',...
        'FontSize',8,...
        'EdgeColor',[1 1 1]);
        %
        subplot(3,2,5);
        plot(D2_Ia, 'r'); hold on;
        plot(D2_Ib, 'b'); hold on;
        plot(D2_Ic, 'g'); hold off;
        xlabel({'Number of samples','(e) D2 Coefficient'},'FontWeight','bold');
        ylabel({'Magnitude'},'FontWeight','bold');
        leg = legend('show', 'Ia', 'Ib', 'Ic');
        set(leg,'Units','pixels',...
        'Orientation','vertical',...
        'location', 'northwest',...
        'Interpreter','none',...
        'FontSize',8,...
        'EdgeColor',[1 1 1]);
        %
        subplot(3,2,6);
        plot(D1_Ia, 'r'); hold on;
        plot(D1_Ib, 'b'); hold on;
        plot(D1_Ic, 'g'); hold off;
        xlabel({'Number of samples','(f) D1 Coefficient'},'FontWeight','bold');
        ylabel({'Magnitude'},'FontWeight','bold');
        leg = legend('show', 'Ia', 'Ib', 'Ic');
        set(leg,'Units','pixels',...
        'Orientation','vertical',...
        'location', 'northwest',...
        'Interpreter','none',...
        'FontSize',8,...
        'EdgeColor',[1 1 1]);
        %
    end
end

== matlab function My_Design/DATA COLLECTION UNIT/DWT ==
  settings: updateMethod=DISCRETE  sampleTime=1e-5
  data: i input; reA4 output; reD4 output; reD3 output; reD2 output; reD1 output; stdA4 output; stdD4 output; stdD3 output; stdD2 output; stdD1 output
function [reA4,reD4,reD3,reD2, reD1,stdA4,stdD4,stdD3,stdD2,stdD1] = DWT(i)
%% CONVERT INPUT DISCRETE SAMPLES TO a 1-D SIGNAL
persistent I;
if isempty(I)
    I = i;
else
    I = [I; i];
end
%%
%% GET 1-D DISCRETE SIGNAL DIRECTLY FROM SAVED FAULTS
[CI,LI] = wavedec(I,4,'db4');
A4 = appcoef(CI,LI,'db4',4);
D4 = detcoef(CI,LI,4);
D3 = detcoef(CI,LI,3);
D2 = detcoef(CI,LI,2);
D1 = detcoef(CI,LI,1);
%% STATISTICAL AND STD CALCULATIONS
Ej_A4 = sum(A4.^2);
Ej_D4 = sum(D4.^2);
Ej_D3 = sum(D3.^2);
Ej_D2 = sum(D2.^2);
Ej_D1 = sum(D1.^2);
E_total = Ej_A4 + Ej_D4 + Ej_D3 + Ej_D2 + Ej_D1;
reA4 = Ej_A4 / E_total;
reD4 = Ej_D4 / E_total;
reD3 = Ej_D3 / E_total;
reD2 = Ej_D2 / E_total;
reD1 = Ej_D1 / E_total;
stdA4 = std(A4);
stdD4 = std(D4);
stdD3 = std(D3);
stdD2 = std(D2);
stdD1 = std(D1);
end

== matlab function My_Design/DATA COLLECTION UNIT/DWT1 ==
  settings: updateMethod=DISCRETE  sampleTime=1e-5
  data: i input; reA4 output; reD4 output; reD3 output; reD2 output; reD1 output; stdA4 output; stdD4 output; stdD3 output; stdD2 output; stdD1 output
function [reA4,reD4,reD3,reD2, reD1,stdA4,stdD4,stdD3,stdD2,stdD1] = DWT(i)
%% CONVERT INPUT DISCRETE SAMPLES TO a 1-D SIGNAL
persistent I;
if isempty(I)
    I = i;
else
    I = [I; i];
end
%%
%% GET 1-D DISCRETE SIGNAL DIRECTLY FROM SAVED FAULTS
[CI,LI] = wavedec(I,4,'db4');
A4 = appcoef(CI,LI,'db4',4);
D4 = detcoef(CI,LI,4);
D3 = detcoef(CI,LI,3);
D2 = detcoef(CI,LI,2);
D1 = detcoef(CI,LI,1);
%% STATISTICAL AND STD CALCULATIONS
Ej_A4 = sum(A4.^2);
Ej_D4 = sum(D4.^2);
Ej_D3 = sum(D3.^2);
Ej_D2 = sum(D2.^2);
Ej_D1 = sum(D1.^2);
E_total = Ej_A4 + Ej_D4 + Ej_D3 + Ej_D2 + Ej_D1;
reA4 = Ej_A4 / E_total;
reD4 = Ej_D4 / E_total;
reD3 = Ej_D3 / E_total;
reD2 = Ej_D2 / E_total;
reD1 = Ej_D1 / E_total;
stdA4 = std(A4);
stdD4 = std(D4);
stdD3 = std(D3);
stdD2 = std(D2);
stdD1 = std(D1);
end

== matlab function My_Design/DATA COLLECTION UNIT/DWT2 ==
  settings: updateMethod=DISCRETE  sampleTime=1e-5
  data: i input; reA4 output; reD4 output; reD3 output; reD2 output; reD1 output; stdA4 output; stdD4 output; stdD3 output; stdD2 output; stdD1 output
function [reA4,reD4,reD3,reD2, reD1,stdA4,stdD4,stdD3,stdD2,stdD1] = DWT(i)
%% CONVERT INPUT DISCRETE SAMPLES TO a 1-D SIGNAL
persistent I;
if isempty(I)
    I = i;
else
    I = [I; i];
end
%%
%% GET 1-D DISCRETE SIGNAL DIRECTLY FROM SAVED FAULTS
[CI,LI] = wavedec(I,4,'db4');
A4 = appcoef(CI,LI,'db4',4);
D4 = detcoef(CI,LI,4);
D3 = detcoef(CI,LI,3);
D2 = detcoef(CI,LI,2);
D1 = detcoef(CI,LI,1);
%% STATISTICAL AND STD CALCULATIONS
Ej_A4 = sum(A4.^2);
Ej_D4 = sum(D4.^2);
Ej_D3 = sum(D3.^2);
Ej_D2 = sum(D2.^2);
Ej_D1 = sum(D1.^2);
E_total = Ej_A4 + Ej_D4 + Ej_D3 + Ej_D2 + Ej_D1;
reA4 = Ej_A4 / E_total;
reD4 = Ej_D4 / E_total;
reD3 = Ej_D3 / E_total;
reD2 = Ej_D2 / E_total;
reD1 = Ej_D1 / E_total;
stdA4 = std(A4);
stdD4 = std(D4);
stdD3 = std(D3);
stdD2 = std(D2);
stdD1 = std(D1);
end

== matlab function My_Design/DIFFERENTIAL RELAY/Intelligence Unit /DWT ==
  settings: updateMethod=DISCRETE  sampleTime=1e-5
  data: i input; reA4 output; reD4 output; reD3 output; reD2 output; reD1 output; stdA4 output; stdD4 output; stdD3 output; stdD2 output; stdD1 output
function [reA4,reD4,reD3,reD2, reD1,stdA4,stdD4,stdD3,stdD2,stdD1] = DWT(i)
%% CONVERT INPUT DISCRETE SAMPLES TO a 1-D SIGNAL
persistent I;
if isempty(I)
    I = i;
else
    I = [I; i];
end
%%
%% GET 1-D DISCRETE SIGNAL DIRECTLY FROM SAVED FAULTS
[CI,LI] = wavedec(I,4,'db4');
A4 = appcoef(CI,LI,'db4',4);
D4 = detcoef(CI,LI,4);
D3 = detcoef(CI,LI,3);
D2 = detcoef(CI,LI,2);
D1 = detcoef(CI,LI,1);
%% STATISTICAL AND RMS CALCULATIONS
Ej_A4 = sum(A4.^2);
Ej_D4 = sum(D4.^2);
Ej_D3 = sum(D3.^2);
Ej_D2 = sum(D2.^2);
Ej_D1 = sum(D1.^2);
E_total = Ej_A4 + Ej_D4 + Ej_D3 + Ej_D2 + Ej_D1;
reA4 = Ej_A4 / E_total;
reD4 = Ej_D4 / E_total;
reD3 = Ej_D3 / E_total;
reD2 = Ej_D2 / E_total;
reD1 = Ej_D1 / E_total;
stdA4 = std(A4);
stdD4 = std(D4);
stdD3 = std(D3);
stdD2 = std(D2);
stdD1 = std(D1);
end

== matlab function My_Design/DIFFERENTIAL RELAY/Intelligence Unit/DWT ==
  settings: updateMethod=DISCRETE  sampleTime=1e-5
  data: i input; reA4 output; reD4 output; reD3 output; reD2 output; reD1 output; stdA4 output; stdD4 output; stdD3 output; stdD2 output; stdD1 output
function [reA4,reD4,reD3,reD2, reD1,stdA4,stdD4,stdD3,stdD2,stdD1] = DWT(i)
%% CONVERT INPUT DISCRETE SAMPLES TO a 1-D SIGNAL
persistent I;
if isempty(I)
    I = i;
else
    I = [I; i];
end
%%
%% GET 1-D DISCRETE SIGNAL DIRECTLY FROM SAVED FAULTS
[CI,LI] = wavedec(I,4,'db4');
A4 = appcoef(CI,LI,'db4',4);
D4 = detcoef(CI,LI,4);
D3 = detcoef(CI,LI,3);
D2 = detcoef(CI,LI,2);
D1 = detcoef(CI,LI,1);
%% STATISTICAL AND RMS CALCULATIONS
Ej_A4 = sum(A4.^2);
Ej_D4 = sum(D4.^2);
Ej_D3 = sum(D3.^2);
Ej_D2 = sum(D2.^2);
Ej_D1 = sum(D1.^2);
E_total = Ej_A4 + Ej_D4 + Ej_D3 + Ej_D2 + Ej_D1;
reA4 = Ej_A4 / E_total;
reD4 = Ej_D4 / E_total;
reD3 = Ej_D3 / E_total;
reD2 = Ej_D2 / E_total;
reD1 = Ej_D1 / E_total;
stdA4 = std(A4);
stdD4 = std(D4);
stdD3 = std(D3);
stdD2 = std(D2);
stdD1 = std(D1);
end

== matlab function My_Design/DIFFERENTIAL RELAY/Intelligence Unit /Decoder ==
  data: anfis input; fault output; target output
function [fault, target] = DECODE(anfis)
%% INTERPRETATING THE RESULTS
%{
    The faults were representated numerically during the preprocessing
    state in Python. This was the represatation
    0 - Inrush condition / Transient current
    1 - Line faultt
    2 - Ground fault
    3 - normal condition / Healthy
%}
%% Give a tolerance of 10 for all faults since it is a practical system
persistent Faulttol;
if isempty(Faulttol)
    Faulttol = 0;
end
target = round(anfis);
if target == 0
    fault = false;
    condition = 'C: External Fault';
    disp(condition);
elseif target == 1
    condition = 'C: Ground Fault';
    disp(condition);
    fault = true;
elseif target == 2
    condition = 'C: Inrush Currents';
    disp(condition);
    fault = false;
elseif target == 3
    condition = 'C: Line Fault';
    disp(condition);
    fault = true;
else
    condition = 'C: Healthy';
    disp(condition);
    fault = false;
end
